simulink model "MultiAgent"  (R2021b)
settings: Solver=ode3  StartTime=0.0  StopTime=160  FixedStep=Ts  RelTol=1e-3
values from neighbouring files (symbols this model uses):
  inner_h = 0.1    [dataset.mat]    (also in initiateVars.m; system_workspace.mat; system_workspace_ayk.mat)
  omega_max_lim = 2500    [dataset.mat]    (also in initiateVars.m; system_workspace.mat; system_workspace_ayk.mat)
  omega_min_lim = 0    [dataset.mat]    (also in initiateVars.m; system_workspace.mat; system_workspace_ayk.mat)
  T_max_lim = 0.495    [dataset.mat]    (also in initiateVars.m = Tp - (Tp - Tm) * sat_lim; system_workspace.mat; system_workspace_ayk.mat)
  T_min_lim = 0.055    [dataset.mat]    (also in initiateVars.m = Tm + (Tp - Tm) * sat_lim; system_workspace.mat; system_workspace_ayk.mat)
  tau_max_lim = 1e-05    [dataset.mat]    (also in initiateVars.m; system_workspace.mat; system_workspace_ayk.mat)
  tau_min_lim = -1e-05    [dataset.mat]    (also in initiateVars.m; system_workspace.mat; system_workspace_ayk.mat)
libraries: slpidlib x4, robotcorelib x2, uavutilslib x2
settings Model: Creator=aykut  LastModifiedBy=fethi
settings SolverCC: AlgebraicLoopSolver=TrustRegion
settings DataIOCC: ReturnWorkspaceOutputs=off
settings DebuggingCC: SFMachineParentedDataDiag=warning  ArithmeticOperatorsInVariantConditions=warning
settings SFSimCC: CustomCodeUndefinedFunction=UseInterfaceOnly

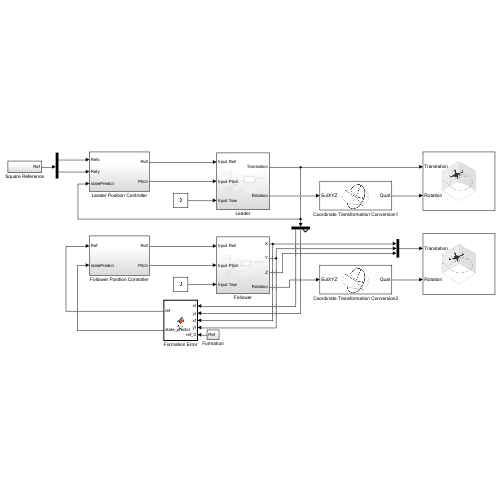
[thumbnail: Simulink's stored preview of the top-level diagram]
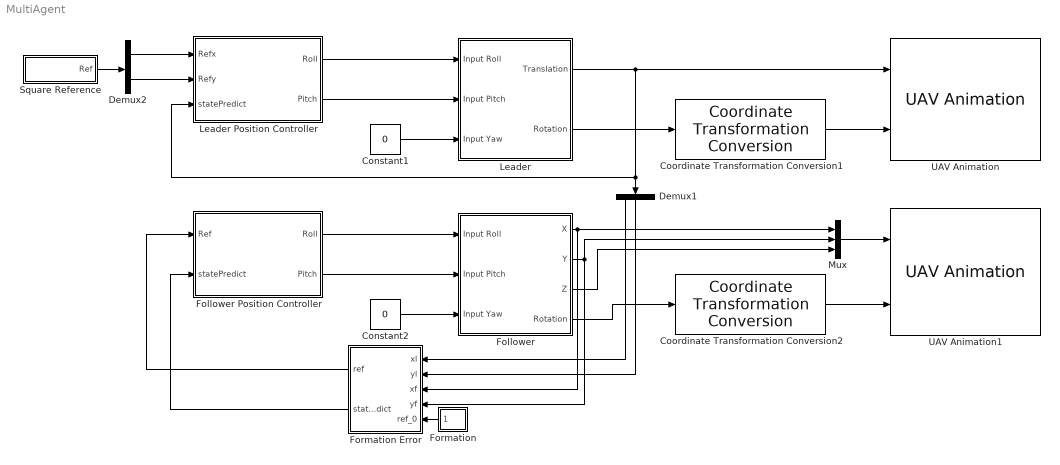
== system MultiAgent ==
  Constant1 : Constant  Value=0
  Constant2 : Constant  Value=0
  Coordinate Transformation Conversion1 : robotcorelib/Coordinate Transformation Conversion  InputRepresentation=Euler Angles  InputEulerSequence=XYZ  ShowTrVecInputPort=on  OutputRepresentation=Quaternion  OutputEulerSequence=ZYX  ShowTrVecOutputPort=on  SimulateUsing=Interpreted execution
      settings: SourceProductBaseCode=NV,RO,RR,UV
  Coordinate Transformation Conversion2 : robotcorelib/Coordinate Transformation Conversion  InputRepresentation=Euler Angles  InputEulerSequence=XYZ  ShowTrVecInputPort=on  OutputRepresentation=Quaternion  OutputEulerSequence=ZYX  ShowTrVecOutputPort=on  SimulateUsing=Interpreted execution
      settings: SourceProductBaseCode=NV,RO,RR,UV
  Demux1 : Demux  Outputs=3
  Demux2 : Demux  Outputs=2
  Follower : Subsystem
  Follower Position Controller : Subsystem
  Formation : Subsystem
  Formation Error : MATLAB Function  TreatAsAtomicUnit=on
  Leader : Subsystem
  Leader Position Controller : Subsystem
  Mux : Mux  Inputs=3
  Square Reference : Subsystem
  UAV Animation : uavutilslib/UAV Animation  UAVType=Multirotor  UAVSize=0.5  InertialZDirection=Up  SampleTime=-1
      settings: SourceProductBaseCode=UV
  UAV Animation1 : uavutilslib/UAV Animation  UAVType=Multirotor  UAVSize=0.5  InertialZDirection=Up  SampleTime=-1
      settings: SourceProductBaseCode=UV
  wires:
  Leader/1(Translation) -> Demux1/1, Leader Position Controller/3(statePredict), UAV Animation/1
  Follower/1(X) -> Formation Error/3(xf), Mux/1
  Follower/2(Y) -> Formation Error/4(yf), Mux/2
  Constant1/1 -> Leader/3(Input Yaw)
  Follower Position Controller/2(Pitch) -> Follower/2(Input Pitch)
  Follower Position Controller/1(Roll) -> Follower/1(Input Roll)
  Constant2/1 -> Follower/3(Input Yaw)
  Leader Position Controller/1(Roll) -> Leader/1(Input Roll)
  Leader Position Controller/2(Pitch) -> Leader/2(Input Pitch)
  Demux2/1 -> Leader Position Controller/1(Refx)
  Demux2/2 -> Leader Position Controller/2(Refy)
  Leader/2(Rotation) -> Coordinate Transformation Conversion1/1
  Coordinate Transformation Conversion1/1 -> UAV Animation/2
  Demux1/1 -> Formation Error/1(xl)
  Demux1/2 -> Formation Error/2(yl)
  Coordinate Transformation Conversion2/1 -> UAV Animation1/2
  Follower/4(Rotation) -> Coordinate Transformation Conversion2/1
  Mux/1 -> UAV Animation1/1
  Square Reference/1(Ref) -> Demux2/1
  Formation Error/1(ref) -> Follower Position Controller/1(Ref)
  Follower/3(Z) -> Mux/3
  Formation Error/2(state_predict) -> Follower Position Controller/2(statePredict)
  Formation/1(Ref) -> Formation Error/5(ref_0)

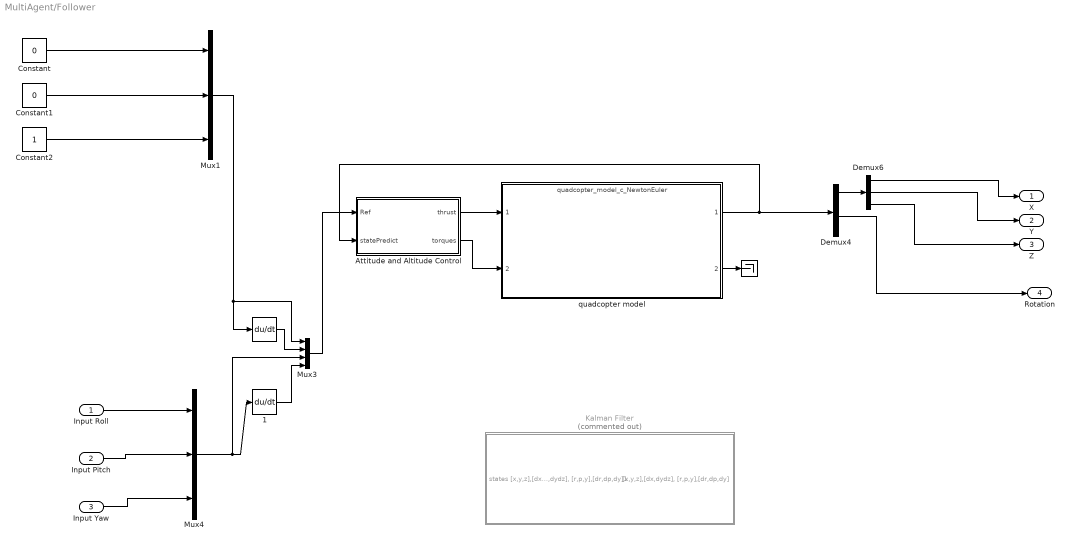
== system MultiAgent/Follower ==
  Input Roll : Inport
  Input Pitch : Inport  Port=2
  Input Yaw : Inport  Port=3
  "   " : Terminator
  "        " : Derivative
  "        1" : Derivative
  Attitude and Altitude Control : Subsystem
  Constant : Constant  Value=0
  Constant1 : Constant  Value=0
  Constant2 : Constant
  Demux4 : Demux  Outputs=[3,3,3,3]
  Demux6 : Demux  Outputs=[1,1,1]
  Kalman Filter : Subsystem  Commented=on
  Mux1 : Mux  Inputs=3
  Mux3 : Mux
  Mux4 : Mux  Inputs=3
  quadcopter model : ModelReference  ModelNameDialog=quadcopter_model_c_NewtonEuler.mdl  SimulationMode=Normal  ModelReferenceVersion=1.355
  X : Outport
  Y : Outport  Port=2
  Z : Outport  Port=3
  Rotation : Outport  Port=4
  wires:
  Mux4/1 -> Mux3/3, "        1"/1
  "        1"/1 -> Mux3/4
  Mux3/1 -> Attitude and Altitude Control/1(Ref)
  Constant/1 -> Mux1/1
  Constant1/1 -> Mux1/2
  "        "/1 -> Mux3/2
  Input Roll/1 -> Mux4/1
  Input Yaw/1 -> Mux4/3
  Constant2/1 -> Mux1/3
  Input Pitch/1 -> Mux4/2
  Mux1/1 -> "        "/1, Mux3/1
  Demux4/1 -> Demux6/1
  quadcopter model/1 -> Attitude and Altitude Control/2(statePredict), Demux4/1
  Attitude and Altitude Control/1(thrust) -> quadcopter model/1
  quadcopter model/2 -> "   "/1
  Attitude and Altitude Control/2(torques) -> quadcopter model/2
  Demux6/1 -> X/1
  Demux6/2 -> Y/1
  Demux6/3 -> Z/1
  Demux4/3 -> Rotation/1

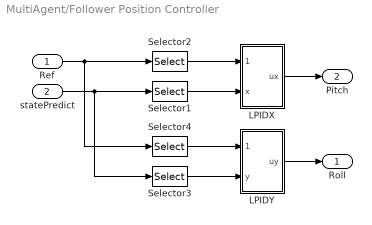
== system MultiAgent/Follower Position Controller ==
  Ref : Inport
  statePredict : Inport  Port=2
  LPIDX : Subsystem
  LPIDY : Subsystem
  Selector1 : Selector  InputPortWidth=2  IndexOptions=Index vector (dialog)  Indices=1  OutputSizes=1
  Selector2 : Selector  InputPortWidth=2  IndexOptions=Index vector (dialog)  Indices=1  OutputSizes=1
  Selector3 : Selector  InputPortWidth=2  IndexOptions=Index vector (dialog)  Indices=2  OutputSizes=1
  Selector4 : Selector  InputPortWidth=2  IndexOptions=Index vector (dialog)  Indices=2  OutputSizes=1
  Roll : Outport  VectorParamsAs1DForOutWhenUnconnected=off
  Pitch : Outport  Port=2  VectorParamsAs1DForOutWhenUnconnected=off
  wires:
  LPIDX/1(ux) -> Pitch/1
  LPIDY/1(uy) -> Roll/1
  statePredict/1 -> Selector1/1, Selector3/1
  Selector3/1 -> LPIDY/2(y)
  Selector1/1 -> LPIDX/2(x)
  Selector2/1 -> LPIDX/1(Refx)
  Ref/1 -> Selector4/1, Selector2/1
  Selector4/1 -> LPIDY/1(Refy)

== system MultiAgent/Formation ==
  Clock : Clock
      settings: Decimation=110
  Mux : Mux  Inputs=2
  Refence Source : MATLAB Function  TreatAsAtomicUnit=on
  Ref : Outport  VectorParamsAs1DForOutWhenUnconnected=off
  wires:
  Refence Source/2(ref_Y) -> Mux/2
  Refence Source/1(ref_X) -> Mux/1
  Mux/1 -> Ref/1
  Clock/1 -> Refence Source/1(timer)

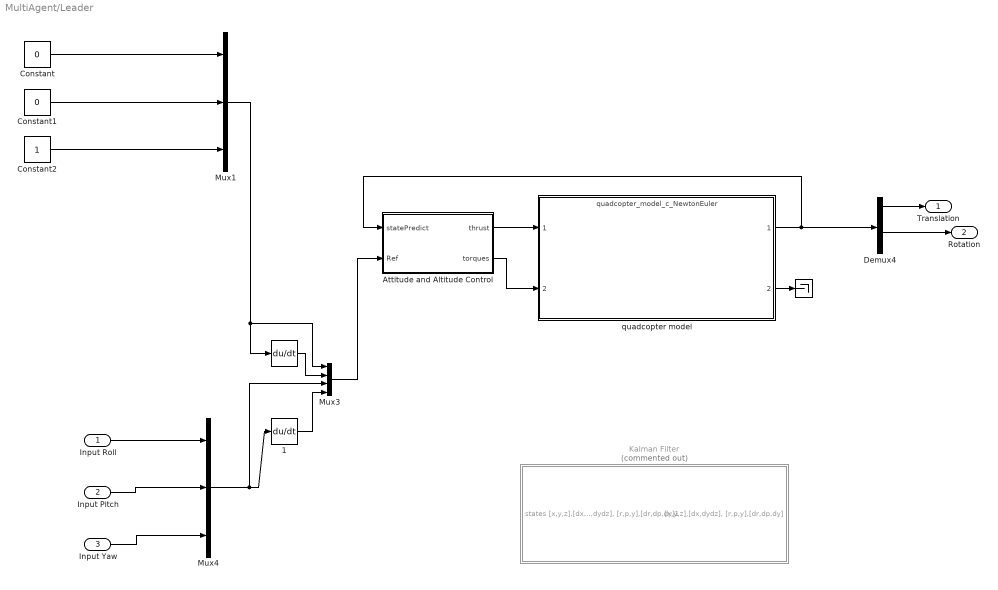
== system MultiAgent/Leader ==
  Input Roll : Inport
  Input Pitch : Inport  Port=2
  Input Yaw : Inport  Port=3
  "   " : Terminator
  "        " : Derivative
  "        1" : Derivative
  Attitude and Altitude Control : Subsystem
  Constant : Constant  Value=0
  Constant1 : Constant  Value=0
  Constant2 : Constant
  Demux4 : Demux  Outputs=[3,3,3,3]
  Kalman Filter : Subsystem  Commented=on
  Mux1 : Mux  Inputs=3
  Mux3 : Mux
  Mux4 : Mux  Inputs=3
  quadcopter model : ModelReference  ModelNameDialog=quadcopter_model_c_NewtonEuler.mdl  SimulationMode=Normal  ModelReferenceVersion=1.355
  Translation : Outport
  Rotation : Outport  Port=2
  wires:
  Attitude and Altitude Control/2(torques) -> quadcopter model/2
  quadcopter model/2 -> "   "/1
  Attitude and Altitude Control/1(thrust) -> quadcopter model/1
  Mux1/1 -> Mux3/1, "        "/1
  Input Pitch/1 -> Mux4/2
  Constant2/1 -> Mux1/3
  Input Yaw/1 -> Mux4/3
  Input Roll/1 -> Mux4/1
  "        "/1 -> Mux3/2
  Constant1/1 -> Mux1/2
  Constant/1 -> Mux1/1
  Mux3/1 -> Attitude and Altitude Control/2(Ref)
  "        1"/1 -> Mux3/4
  Mux4/1 -> "        1"/1, Mux3/3
  quadcopter model/1 -> Attitude and Altitude Control/1(statePredict), Demux4/1
  Demux4/1 -> Translation/1
  Demux4/3 -> Rotation/1

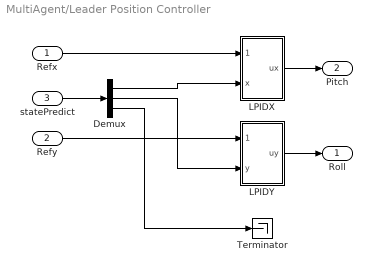
== system MultiAgent/Leader Position Controller ==
  Refx : Inport
  Refy : Inport  Port=2
  statePredict : Inport  Port=3
  Demux : Demux  Outputs=3
  LPIDX : Subsystem
  LPIDY : Subsystem
  Terminator : Terminator
  Roll : Outport  VectorParamsAs1DForOutWhenUnconnected=off
  Pitch : Outport  Port=2  VectorParamsAs1DForOutWhenUnconnected=off
  wires:
  Refx/1 -> LPIDX/1(Refx)
  Refy/1 -> LPIDY/1(Refy)
  LPIDY/1(uy) -> Roll/1
  LPIDX/1(ux) -> Pitch/1
  statePredict/1 -> Demux/1
  Demux/1 -> LPIDX/2(x)
  Demux/2 -> LPIDY/2(y)
  Demux/3 -> Terminator/1

== system MultiAgent/Square Reference ==
  Clock : Clock
      settings: Decimation=110
  Mux : Mux  Inputs=2
  Refence Source : MATLAB Function  TreatAsAtomicUnit=on
  Ref : Outport  VectorParamsAs1DForOutWhenUnconnected=off
  wires:
  Clock/1 -> Refence Source/1(timer)
  Mux/1 -> Ref/1
  Refence Source/1(ref_X) -> Mux/1
  Refence Source/2(ref_Y) -> Mux/2

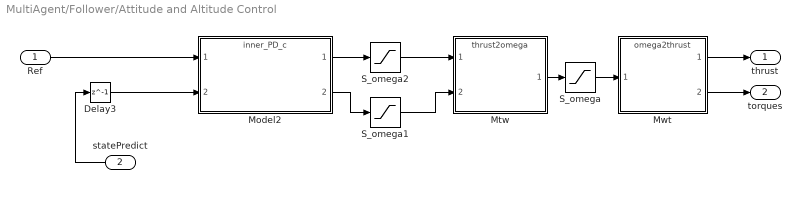
== system MultiAgent/Follower/Attitude and Altitude Control ==
  Ref : Inport
  statePredict : Inport  Port=2
  Delay3 : Delay  DelayLength=1  InitialCondition=0  SampleTime=inner_h
  Model2 : ModelReference  ModelNameDialog=inner_PD_c.mdl  SimulationMode=Normal  ModelReferenceVersion=1.90
  Mtw : ModelReference  ModelNameDialog=thrust2omega.mdl  SimulationMode=Normal  ModelReferenceVersion=1.7
  Mwt : ModelReference  ModelNameDialog=omega2thrust.mdl  SimulationMode=Normal  ModelReferenceVersion=1.7
  S_omega : Saturate  UpperLimit=omega_max_lim  LowerLimit=omega_min_lim
  S_omega1 : Saturate  UpperLimit=tau_max_lim  LowerLimit=tau_min_lim
  S_omega2 : Saturate  UpperLimit=T_max_lim  LowerLimit=T_min_lim
  thrust : Outport  VectorParamsAs1DForOutWhenUnconnected=off
  torques : Outport  Port=2  VectorParamsAs1DForOutWhenUnconnected=off
  wires:
  S_omega/1 -> Mwt/1
  S_omega1/1 -> Mtw/2
  S_omega2/1 -> Mtw/1
  Mtw/1 -> S_omega/1
  Model2/1 -> S_omega2/1
  Mwt/1 -> thrust/1
  Model2/2 -> S_omega1/1
  Delay3/1 -> Model2/2
  Ref/1 -> Model2/1
  Mwt/2 -> torques/1
  statePredict/1 -> Delay3/1

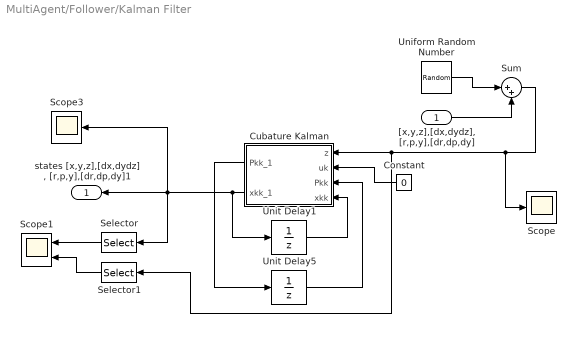
== system MultiAgent/Follower/Kalman Filter ==
  "[x,y,z],[dx,dydz], [r,p,y],[dr,dp,dy]" : Inport
  Constant : Constant  Value=0
  Cubature Kalman : MATLAB Function  TreatAsAtomicUnit=on
  Scope : Scope
  Scope1 : Scope  NumInputPorts=2
  Scope3 : Scope
  Selector : Selector  InputPortWidth=12  IndexOptions=Index vector (dialog)  Indices=[3]  OutputSizes=1
  Selector1 : Selector  InputPortWidth=12  IndexOptions=Index vector (dialog)  Indices=[3]  OutputSizes=1
  Sum : Sum  Inputs=|++
  Uniform Random Number : UniformRandomNumber  Minimum=-0.001  Maximum=0.001  SampleTime=0.1
  Unit Delay1 : UnitDelay  InitialCondition=[0 0 0 0 0 0 0 0 0 0 0 0]  SampleTime=-1  HasFrameUpgradeWarning=on
  Unit Delay5 : UnitDelay  InitialCondition=eye(12)*10^-3  SampleTime=-1  HasFrameUpgradeWarning=on
  "states [x,y,z],[dx,dydz], [r,p,y],[dr,dp,dy]1" : Outport  PortDimensions=12  VectorParamsAs1DForOutWhenUnconnected=off
  wires:
  Unit Delay5/1 -> Cubature Kalman/3(Pkk)
  Cubature Kalman/1(Pkk_1) -> Unit Delay5/1
  Constant/1 -> Cubature Kalman/2(uk)
  Cubature Kalman/2(xkk_1) -> Selector/1, "states [x,y,z],[dx,dydz], [r,p,y],[dr,dp,dy]1"/1, Scope3/1, Unit Delay1/1
  Unit Delay1/1 -> Cubature Kalman/4(xkk)
  Selector/1 -> Scope1/1
  Selector1/1 -> Scope1/2
  Sum/1 -> Selector1/1, Cubature Kalman/1(z), Scope/1
  Uniform Random Number/1 -> Sum/1
  "[x,y,z],[dx,dydz], [r,p,y],[dr,dp,dy]"/1 -> Sum/2

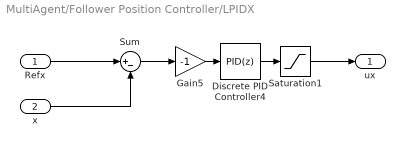
== system MultiAgent/Follower Position Controller/LPIDX ==
  Refx : Inport
  x : Inport  Port=2
  Discrete PID Controller4 : slpidlib/PID Controller  Controller=PID  Form=Parallel  TimeDomain=Discrete-time  UseExternalTs=off  SampleTime=-1  IntegratorMethod=Forward Euler  FilterMethod=Forward Euler  ControllerParametersSource=internal  P=-0.034  I=-8.37942170328314e-06  D=-0.0838262219971284  UseFilter=on  N=16.4387565401463  TunerSelectOption=Transfer Function Based (PID Tuner App)  InitialConditionSource=internal  InitialConditionForIntegrator=0  InitialConditionForFilter=0  DifferentiatorICPrevScaledInput=0  ExternalReset=none  TrackingMode=off  Kt=1  LimitOutput=off  SatLimitsSource=internal  UpperSaturationLimit=inf  LowerSaturationLimit=-inf  LinearizeAsGain=off  AntiWindupMode=none  Kb=1  POutMin=[]  POutMax=[]  IOutMin=[]  IOutMax=[]  DOutMin=[]  DOutMax=[]  NOutMin=[]  NOutMax=[]  SumOutMin=[]  SumOutMax=[]  SaturationOutMin=[]  SaturationOutMax=[]  PParamMin=[]  PParamMax=[]  IParamMin=[]  IParamMax=[]  DParamMin=[]  DParamMax=[]  NParamMin=[]  NParamMax=[]  KbParamMin=[]  KbParamMax=[]  KtParamMin=[]  KtParamMax=[]  KbOutMin=[]  KbOutMax=[]  KtOutMin=[]  KtOutMax=[]  IntegratorOutMin=[]  IntegratorOutMax=[]  FilterOutMin=[]  FilterOutMax=[]  SumI1OutMin=[]  SumI1OutMax=[]  SumI2OutMin=[]  SumI2OutMax=[]  SumI3OutMin=[]  SumI3OutMax=[]  SumI4OutMin=[]  SumI4OutMax=[]  SumDOutMin=[]  SumDOutMax=[]  DifferentiatorOutMin=[]  DifferentiatorOutMax=[]  FilterDiffOutCoefMin=[]  FilterDiffOutCoefMax=[]  ReciprocalOutMin=[]  ReciprocalOutMax=[]  SumDenOutMin=[]  SumDenOutMax=[]  SumNumOutMin=[]  SumNumOutMax=[]  DivideOutMin=[]  DivideOutMax=[]  UdiffTsProdOutMin=[]  UdiffTsProdOutMax=[]  NTsProdOutMin=[]  NTsProdOutMax=[]  UintegralTsProdOutMin=[]  UintegralTsProdOutMax=[]  UngainTsProdOutMin=[]  UngainTsProdOutMax=[]  IntegratorContinuousStateAttributes=''  IntegratorStateMustResolveToSignalObject=off  IntegratorRTWStateStorageClass=Auto  FilterContinuousStateAttributes=''  FilterStateMustResolveToSignalObject=off  FilterRTWStateStorageClass=Auto  ParallelPVariant=InternalParameters  IdealPVariant=Disabled  IVariant=InternalParameters  DVariant=InternalParameters  IntegratorVariant=Discrete  SatVariant=Disabled  AWVariant=Passthrough  PCopyVariant=Disabled  TRVariant=Disabled  FdbkBlocksVariant=Forward  IdealPFdbkVariant=Disabled  SatFdbkVariant=Disabled  DerivativeFilterVariant=ForwardEulerFilter  NVariant=InternalParameters  NCopyVariant=Disabled  FilterICVariant=InternalICsFilter  IntegratorICVariant=InternalICs  ExternalResetVariant=Disabled  TRSumVariant=Passthrough  SumFdbkVariant=Disabled  SumVariant=Sum_PID  TsampFilterVariant=InternalTs  TsampNgainVariant=Passthrough  TsampIntegralVariant=Passthrough  ExternalSaturationOutDataTypeStr=Inherit: Same as second input
  Gain5 : Gain  Gain=-1
  Saturation1 : Saturate  UpperLimit=pi/18  LowerLimit=-pi/18
  Sum : Sum  Inputs=|+-
  ux : Outport  VectorParamsAs1DForOutWhenUnconnected=off
  wires:
  Saturation1/1 -> ux/1
  Sum/1 -> Gain5/1
  Discrete PID Controller4/1 -> Saturation1/1
  x/1 -> Sum/2
  Refx/1 -> Sum/1
  Gain5/1 -> Discrete PID Controller4/1

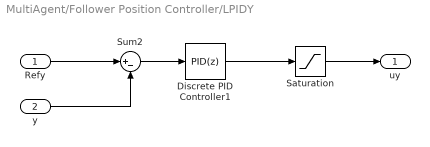
== system MultiAgent/Follower Position Controller/LPIDY ==
  Refy : Inport
  y : Inport  Port=2
  Discrete PID Controller1 : slpidlib/PID Controller  Controller=PID  Form=Parallel  TimeDomain=Discrete-time  UseExternalTs=off  SampleTime=-1  IntegratorMethod=Forward Euler  FilterMethod=Forward Euler  ControllerParametersSource=internal  P=-0.034  I=-8.37942170328314e-06  D=-0.0838262219971284  UseFilter=on  N=16.4387565401463  TunerSelectOption=Transfer Function Based (PID Tuner App)  InitialConditionSource=internal  InitialConditionForIntegrator=0  InitialConditionForFilter=0  DifferentiatorICPrevScaledInput=0  ExternalReset=none  TrackingMode=off  Kt=1  LimitOutput=off  SatLimitsSource=internal  UpperSaturationLimit=inf  LowerSaturationLimit=-inf  LinearizeAsGain=off  AntiWindupMode=none  Kb=1  POutMin=[]  POutMax=[]  IOutMin=[]  IOutMax=[]  DOutMin=[]  DOutMax=[]  NOutMin=[]  NOutMax=[]  SumOutMin=[]  SumOutMax=[]  SaturationOutMin=[]  SaturationOutMax=[]  PParamMin=[]  PParamMax=[]  IParamMin=[]  IParamMax=[]  DParamMin=[]  DParamMax=[]  NParamMin=[]  NParamMax=[]  KbParamMin=[]  KbParamMax=[]  KtParamMin=[]  KtParamMax=[]  KbOutMin=[]  KbOutMax=[]  KtOutMin=[]  KtOutMax=[]  IntegratorOutMin=[]  IntegratorOutMax=[]  FilterOutMin=[]  FilterOutMax=[]  SumI1OutMin=[]  SumI1OutMax=[]  SumI2OutMin=[]  SumI2OutMax=[]  SumI3OutMin=[]  SumI3OutMax=[]  SumI4OutMin=[]  SumI4OutMax=[]  SumDOutMin=[]  SumDOutMax=[]  DifferentiatorOutMin=[]  DifferentiatorOutMax=[]  FilterDiffOutCoefMin=[]  FilterDiffOutCoefMax=[]  ReciprocalOutMin=[]  ReciprocalOutMax=[]  SumDenOutMin=[]  SumDenOutMax=[]  SumNumOutMin=[]  SumNumOutMax=[]  DivideOutMin=[]  DivideOutMax=[]  UdiffTsProdOutMin=[]  UdiffTsProdOutMax=[]  NTsProdOutMin=[]  NTsProdOutMax=[]  UintegralTsProdOutMin=[]  UintegralTsProdOutMax=[]  UngainTsProdOutMin=[]  UngainTsProdOutMax=[]  IntegratorContinuousStateAttributes=''  IntegratorStateMustResolveToSignalObject=off  IntegratorRTWStateStorageClass=Auto  FilterContinuousStateAttributes=''  FilterStateMustResolveToSignalObject=off  FilterRTWStateStorageClass=Auto  ParallelPVariant=InternalParameters  IdealPVariant=Disabled  IVariant=InternalParameters  DVariant=InternalParameters  IntegratorVariant=Discrete  SatVariant=Disabled  AWVariant=Passthrough  PCopyVariant=Disabled  TRVariant=Disabled  FdbkBlocksVariant=Forward  IdealPFdbkVariant=Disabled  SatFdbkVariant=Disabled  DerivativeFilterVariant=ForwardEulerFilter  NVariant=InternalParameters  NCopyVariant=Disabled  FilterICVariant=InternalICsFilter  IntegratorICVariant=InternalICs  ExternalResetVariant=Disabled  TRSumVariant=Passthrough  SumFdbkVariant=Disabled  SumVariant=Sum_PID  TsampFilterVariant=InternalTs  TsampNgainVariant=Passthrough  TsampIntegralVariant=Passthrough  ExternalSaturationOutDataTypeStr=Inherit: Same as second input
  Saturation : Saturate  UpperLimit=pi/18  LowerLimit=-pi/18
  Sum2 : Sum  Inputs=|+-
  uy : Outport  VectorParamsAs1DForOutWhenUnconnected=off
  wires:
  Saturation/1 -> uy/1
  y/1 -> Sum2/2
  Refy/1 -> Sum2/1
  Discrete PID Controller1/1 -> Saturation/1
  Sum2/1 -> Discrete PID Controller1/1

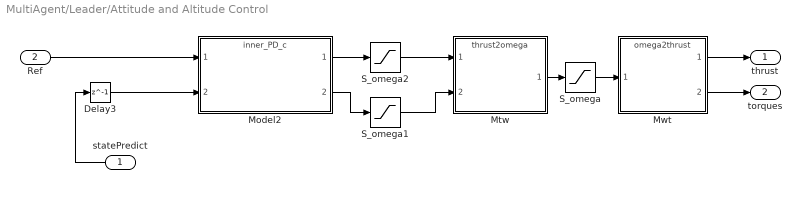
== system MultiAgent/Leader/Attitude and Altitude Control ==
  statePredict : Inport
  Ref : Inport  Port=2
  Delay3 : Delay  DelayLength=1  InitialCondition=0  SampleTime=inner_h
  Model2 : ModelReference  ModelNameDialog=inner_PD_c.mdl  SimulationMode=Normal  ModelReferenceVersion=1.90
  Mtw : ModelReference  ModelNameDialog=thrust2omega.mdl  SimulationMode=Normal  ModelReferenceVersion=1.7
  Mwt : ModelReference  ModelNameDialog=omega2thrust.mdl  SimulationMode=Normal  ModelReferenceVersion=1.7
  S_omega : Saturate  UpperLimit=omega_max_lim  LowerLimit=omega_min_lim
  S_omega1 : Saturate  UpperLimit=tau_max_lim  LowerLimit=tau_min_lim
  S_omega2 : Saturate  UpperLimit=T_max_lim  LowerLimit=T_min_lim
  thrust : Outport  VectorParamsAs1DForOutWhenUnconnected=off
  torques : Outport  Port=2  VectorParamsAs1DForOutWhenUnconnected=off
  wires:
  statePredict/1 -> Delay3/1
  Mwt/2 -> torques/1
  Ref/1 -> Model2/1
  Delay3/1 -> Model2/2
  Model2/2 -> S_omega1/1
  Mwt/1 -> thrust/1
  Model2/1 -> S_omega2/1
  Mtw/1 -> S_omega/1
  S_omega2/1 -> Mtw/1
  S_omega1/1 -> Mtw/2
  S_omega/1 -> Mwt/1

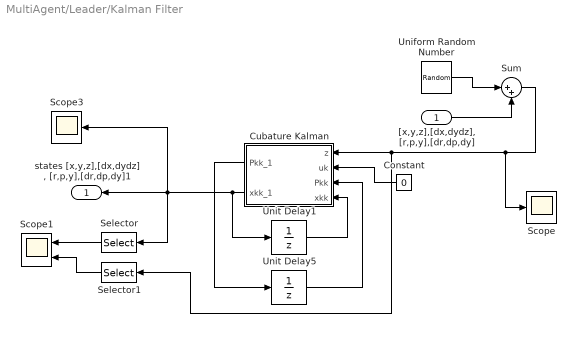
== system MultiAgent/Leader/Kalman Filter ==
  "[x,y,z],[dx,dydz], [r,p,y],[dr,dp,dy]" : Inport
  Constant : Constant  Value=0
  Cubature Kalman : MATLAB Function  TreatAsAtomicUnit=on
  Scope : Scope
  Scope1 : Scope  NumInputPorts=2
  Scope3 : Scope
  Selector : Selector  InputPortWidth=12  IndexOptions=Index vector (dialog)  Indices=[3]  OutputSizes=1
  Selector1 : Selector  InputPortWidth=12  IndexOptions=Index vector (dialog)  Indices=[3]  OutputSizes=1
  Sum : Sum  Inputs=|++
  Uniform Random Number : UniformRandomNumber  Minimum=-0.001  Maximum=0.001  SampleTime=0.1
  Unit Delay1 : UnitDelay  InitialCondition=[0 0 0 0 0 0 0 0 0 0 0 0]  SampleTime=-1  HasFrameUpgradeWarning=on
  Unit Delay5 : UnitDelay  InitialCondition=eye(12)*10^-3  SampleTime=-1  HasFrameUpgradeWarning=on
  "states [x,y,z],[dx,dydz], [r,p,y],[dr,dp,dy]1" : Outport  PortDimensions=12  VectorParamsAs1DForOutWhenUnconnected=off
  wires:
  "[x,y,z],[dx,dydz], [r,p,y],[dr,dp,dy]"/1 -> Sum/2
  Uniform Random Number/1 -> Sum/1
  Sum/1 -> Scope/1, Cubature Kalman/1(z), Selector1/1
  Selector1/1 -> Scope1/2
  Selector/1 -> Scope1/1
  Unit Delay1/1 -> Cubature Kalman/4(xkk)
  Cubature Kalman/2(xkk_1) -> Unit Delay1/1, Scope3/1, "states [x,y,z],[dx,dydz], [r,p,y],[dr,dp,dy]1"/1, Selector/1
  Constant/1 -> Cubature Kalman/2(uk)
  Cubature Kalman/1(Pkk_1) -> Unit Delay5/1
  Unit Delay5/1 -> Cubature Kalman/3(Pkk)

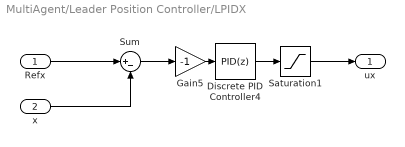
== system MultiAgent/Leader Position Controller/LPIDX ==
  Refx : Inport
  x : Inport  Port=2
  Discrete PID Controller4 : slpidlib/PID Controller  Controller=PID  Form=Parallel  TimeDomain=Discrete-time  UseExternalTs=off  SampleTime=-1  IntegratorMethod=Forward Euler  FilterMethod=Forward Euler  ControllerParametersSource=internal  P=-0.034  I=-7.00942170328314e-06  D=-0.0838262219971284  UseFilter=on  N=16.4387565401463  TunerSelectOption=Transfer Function Based (PID Tuner App)  InitialConditionSource=internal  InitialConditionForIntegrator=0  InitialConditionForFilter=0  DifferentiatorICPrevScaledInput=0  ExternalReset=none  TrackingMode=off  Kt=1  LimitOutput=off  SatLimitsSource=internal  UpperSaturationLimit=inf  LowerSaturationLimit=-inf  LinearizeAsGain=off  AntiWindupMode=none  Kb=1  POutMin=[]  POutMax=[]  IOutMin=[]  IOutMax=[]  DOutMin=[]  DOutMax=[]  NOutMin=[]  NOutMax=[]  SumOutMin=[]  SumOutMax=[]  SaturationOutMin=[]  SaturationOutMax=[]  PParamMin=[]  PParamMax=[]  IParamMin=[]  IParamMax=[]  DParamMin=[]  DParamMax=[]  NParamMin=[]  NParamMax=[]  KbParamMin=[]  KbParamMax=[]  KtParamMin=[]  KtParamMax=[]  KbOutMin=[]  KbOutMax=[]  KtOutMin=[]  KtOutMax=[]  IntegratorOutMin=[]  IntegratorOutMax=[]  FilterOutMin=[]  FilterOutMax=[]  SumI1OutMin=[]  SumI1OutMax=[]  SumI2OutMin=[]  SumI2OutMax=[]  SumI3OutMin=[]  SumI3OutMax=[]  SumI4OutMin=[]  SumI4OutMax=[]  SumDOutMin=[]  SumDOutMax=[]  DifferentiatorOutMin=[]  DifferentiatorOutMax=[]  FilterDiffOutCoefMin=[]  FilterDiffOutCoefMax=[]  ReciprocalOutMin=[]  ReciprocalOutMax=[]  SumDenOutMin=[]  SumDenOutMax=[]  SumNumOutMin=[]  SumNumOutMax=[]  DivideOutMin=[]  DivideOutMax=[]  UdiffTsProdOutMin=[]  UdiffTsProdOutMax=[]  NTsProdOutMin=[]  NTsProdOutMax=[]  UintegralTsProdOutMin=[]  UintegralTsProdOutMax=[]  UngainTsProdOutMin=[]  UngainTsProdOutMax=[]  IntegratorContinuousStateAttributes=''  IntegratorStateMustResolveToSignalObject=off  IntegratorRTWStateStorageClass=Auto  FilterContinuousStateAttributes=''  FilterStateMustResolveToSignalObject=off  FilterRTWStateStorageClass=Auto  ParallelPVariant=InternalParameters  IdealPVariant=Disabled  IVariant=InternalParameters  DVariant=InternalParameters  IntegratorVariant=Discrete  SatVariant=Disabled  AWVariant=Passthrough  PCopyVariant=Disabled  TRVariant=Disabled  FdbkBlocksVariant=Forward  IdealPFdbkVariant=Disabled  SatFdbkVariant=Disabled  DerivativeFilterVariant=ForwardEulerFilter  NVariant=InternalParameters  NCopyVariant=Disabled  FilterICVariant=InternalICsFilter  IntegratorICVariant=InternalICs  ExternalResetVariant=Disabled  TRSumVariant=Passthrough  SumFdbkVariant=Disabled  SumVariant=Sum_PID  TsampFilterVariant=InternalTs  TsampNgainVariant=Passthrough  TsampIntegralVariant=Passthrough  ExternalSaturationOutDataTypeStr=Inherit: Same as second input
  Gain5 : Gain  Gain=-1
  Saturation1 : Saturate  UpperLimit=pi/18  LowerLimit=-pi/18
  Sum : Sum  Inputs=|+-
  ux : Outport  VectorParamsAs1DForOutWhenUnconnected=off
  wires:
  Refx/1 -> Sum/1
  x/1 -> Sum/2
  Discrete PID Controller4/1 -> Saturation1/1
  Sum/1 -> Gain5/1
  Gain5/1 -> Discrete PID Controller4/1
  Saturation1/1 -> ux/1

== system MultiAgent/Leader Position Controller/LPIDY ==
  Refy : Inport
  y : Inport  Port=2
  Discrete PID Controller1 : slpidlib/PID Controller  Controller=PID  Form=Parallel  TimeDomain=Discrete-time  UseExternalTs=off  SampleTime=-1  IntegratorMethod=Forward Euler  FilterMethod=Forward Euler  ControllerParametersSource=internal  P=-0.034  I=-7.00942170328314e-06  D=-0.0838262219971284  UseFilter=on  N=16.4387565401463  TunerSelectOption=Transfer Function Based (PID Tuner App)  InitialConditionSource=internal  InitialConditionForIntegrator=0  InitialConditionForFilter=0  DifferentiatorICPrevScaledInput=0  ExternalReset=none  TrackingMode=off  Kt=1  LimitOutput=off  SatLimitsSource=internal  UpperSaturationLimit=inf  LowerSaturationLimit=-inf  LinearizeAsGain=off  AntiWindupMode=none  Kb=1  POutMin=[]  POutMax=[]  IOutMin=[]  IOutMax=[]  DOutMin=[]  DOutMax=[]  NOutMin=[]  NOutMax=[]  SumOutMin=[]  SumOutMax=[]  SaturationOutMin=[]  SaturationOutMax=[]  PParamMin=[]  PParamMax=[]  IParamMin=[]  IParamMax=[]  DParamMin=[]  DParamMax=[]  NParamMin=[]  NParamMax=[]  KbParamMin=[]  KbParamMax=[]  KtParamMin=[]  KtParamMax=[]  KbOutMin=[]  KbOutMax=[]  KtOutMin=[]  KtOutMax=[]  IntegratorOutMin=[]  IntegratorOutMax=[]  FilterOutMin=[]  FilterOutMax=[]  SumI1OutMin=[]  SumI1OutMax=[]  SumI2OutMin=[]  SumI2OutMax=[]  SumI3OutMin=[]  SumI3OutMax=[]  SumI4OutMin=[]  SumI4OutMax=[]  SumDOutMin=[]  SumDOutMax=[]  DifferentiatorOutMin=[]  DifferentiatorOutMax=[]  FilterDiffOutCoefMin=[]  FilterDiffOutCoefMax=[]  ReciprocalOutMin=[]  ReciprocalOutMax=[]  SumDenOutMin=[]  SumDenOutMax=[]  SumNumOutMin=[]  SumNumOutMax=[]  DivideOutMin=[]  DivideOutMax=[]  UdiffTsProdOutMin=[]  UdiffTsProdOutMax=[]  NTsProdOutMin=[]  NTsProdOutMax=[]  UintegralTsProdOutMin=[]  UintegralTsProdOutMax=[]  UngainTsProdOutMin=[]  UngainTsProdOutMax=[]  IntegratorContinuousStateAttributes=''  IntegratorStateMustResolveToSignalObject=off  IntegratorRTWStateStorageClass=Auto  FilterContinuousStateAttributes=''  FilterStateMustResolveToSignalObject=off  FilterRTWStateStorageClass=Auto  ParallelPVariant=InternalParameters  IdealPVariant=Disabled  IVariant=InternalParameters  DVariant=InternalParameters  IntegratorVariant=Discrete  SatVariant=Disabled  AWVariant=Passthrough  PCopyVariant=Disabled  TRVariant=Disabled  FdbkBlocksVariant=Forward  IdealPFdbkVariant=Disabled  SatFdbkVariant=Disabled  DerivativeFilterVariant=ForwardEulerFilter  NVariant=InternalParameters  NCopyVariant=Disabled  FilterICVariant=InternalICsFilter  IntegratorICVariant=InternalICs  ExternalResetVariant=Disabled  TRSumVariant=Passthrough  SumFdbkVariant=Disabled  SumVariant=Sum_PID  TsampFilterVariant=InternalTs  TsampNgainVariant=Passthrough  TsampIntegralVariant=Passthrough  ExternalSaturationOutDataTypeStr=Inherit: Same as second input
  Saturation : Saturate  UpperLimit=pi/18  LowerLimit=-pi/18
  Sum2 : Sum  Inputs=|+-
  uy : Outport  VectorParamsAs1DForOutWhenUnconnected=off
  wires:
  Refy/1 -> Sum2/1
  y/1 -> Sum2/2
  Sum2/1 -> Discrete PID Controller1/1
  Saturation/1 -> uy/1
  Discrete PID Controller1/1 -> Saturation/1

== matlab function MultiAgent/Leader/Kalman Filter/Cubature Kalman ==
  data: Pkk_1 output; z input; uk input; Pkk input; xkk input; xkk_1 output
function [Pkk_1, xkk_1]   = fcn(z, uk, Pkk, xkk)

%% Model
A = 1;
B = 0;

%% Covariances
Q = diag([0.1 0.1 0.1 0.1 0.1 0.1 0.1 0.1 0.1 0.1 0.1 0.1])*100;
R = 0.01;   
% gyro = z(4:6);
% delta = [1*(gyro'-xkk(4:6));0;0;0;0];
% z1 = [z(1:3)' - xkk(1:3); z(1:3)' - xkk(1:3); z(7)];  
%% Cubature Kalman Predict
xkk1 = A*xkk ;
Pkk1 = A*Pkk*A' + Q; 

%% Cubature Kalman Update
%%%========================================================================
%%% Genrate a set of Cubature Points
%%%========================================================================

nx = 12; % state vector dimension

nPts = 2*nx;   % No. of Cubature Points

CPtArray = sqrt(nPts/2)*[eye(nx) -eye(nx)];

%%%========================================================================
%%% find the square-root of Pkk1 using Singular Value Decomposition (SVD)
%%%========================================================================

Pkk1 = 0.5*(Pkk1+Pkk1'); % make Pkk1 to be symmetric (Property of a covariance matrix !)

[U, S, V] =  svd(Pkk1);

Skk1 = 0.5*(U+V)*sqrt(S);

%%%========================================================================

Xi =  repmat(xkk1,1,nPts) + Skk1*CPtArray;

% Zi = Zi1(1,:);
% Zi = cartpend(Xi,uk, Zi1);
% bias = [0.00017;0.00017;0.00017;0.00076;0.00076;0.00076;0.001]; 
% bias = repmat(bias,1,14);
Zi = Xi;
% Zi = Zi1';

    

zkk1 = sum(Zi,2)/nPts;      % predicted Measurement

X = (Xi-repmat(xkk1,1,nPts))/sqrt(nPts);
    
Z = (Zi-repmat(zkk1,1,nPts))/sqrt(nPts);  

Pzz = Z*Z'+ R; % Innovations Covariance

Pxz = X*Z'; % cross-covariance
    
G = Pxz*pinv(Pzz);         % Cubature Kalman Gain  
    
xkk_1 = xkk1 + G*(z - zkk1);  

Pkk_1 = Pkk1 - G*Pzz*G';

== matlab function MultiAgent/Follower/Kalman Filter/Cubature Kalman ==
  data: Pkk_1 output; z input; uk input; Pkk input; xkk input; xkk_1 output
function [Pkk_1, xkk_1]   = fcn(z, uk, Pkk, xkk)

%% Model
A = 1;
B = 0;

%% Covariances
Q = diag([0.1 0.1 0.1 0.1 0.1 0.1 0.1 0.1 0.1 0.1 0.1 0.1])*100;
R = 0.01;   
% gyro = z(4:6);
% delta = [1*(gyro'-xkk(4:6));0;0;0;0];
% z1 = [z(1:3)' - xkk(1:3); z(1:3)' - xkk(1:3); z(7)];  
%% Cubature Kalman Predict
xkk1 = A*xkk ;
Pkk1 = A*Pkk*A' + Q; 

%% Cubature Kalman Update
%%%========================================================================
%%% Genrate a set of Cubature Points
%%%========================================================================

nx = 12; % state vector dimension

nPts = 2*nx;   % No. of Cubature Points

CPtArray = sqrt(nPts/2)*[eye(nx) -eye(nx)];

%%%========================================================================
%%% find the square-root of Pkk1 using Singular Value Decomposition (SVD)
%%%========================================================================

Pkk1 = 0.5*(Pkk1+Pkk1'); % make Pkk1 to be symmetric (Property of a covariance matrix !)

[U, S, V] =  svd(Pkk1);

Skk1 = 0.5*(U+V)*sqrt(S);

%%%========================================================================

Xi =  repmat(xkk1,1,nPts) + Skk1*CPtArray;

% Zi = Zi1(1,:);
% Zi = cartpend(Xi,uk, Zi1);
% bias = [0.00017;0.00017;0.00017;0.00076;0.00076;0.00076;0.001]; 
% bias = repmat(bias,1,14);
Zi = Xi;
% Zi = Zi1';

    

zkk1 = sum(Zi,2)/nPts;      % predicted Measurement

X = (Xi-repmat(xkk1,1,nPts))/sqrt(nPts);
    
Z = (Zi-repmat(zkk1,1,nPts))/sqrt(nPts);  

Pzz = Z*Z'+ R; % Innovations Covariance

Pxz = X*Z'; % cross-covariance
    
G = Pxz*pinv(Pzz);         % Cubature Kalman Gain  
    
xkk_1 = xkk1 + G*(z - zkk1);  

Pkk_1 = Pkk1 - G*Pzz*G';

== matlab function MultiAgent/Formation/Refence Source ==
  data: timer input; ref_X output; ref_Y output
function [ref_X,ref_Y] = fcn(timer)

if timer > 0 && timer < 30
    ref_X = 1;
    ref_Y = 1;

elseif timer >= 30 && timer < 50
    ref_X = -1;
    ref_Y = 1;    
  
elseif timer >= 50 && timer < 70
    ref_X = -1;
    ref_Y = -1;  

elseif timer >= 70 && timer < 90
    ref_X = 1;
    ref_Y = -1; 
    
elseif timer >= 90 && timer < 120
    ref_X = 1;
    ref_Y = 1;
else
    ref_X = 1;
    ref_Y = 1;
end

== matlab function MultiAgent/Formation Error ==
  data: ref output; xl input; yl input; xf input; yf input; state_predict output; ref_0 input
function [ref, state_predict]= fcn(xl,yl,xf,yf, ref_0)
yawl = 0;
dx = -(xl - xf)*cosd(yawl) - (yl - yf)*sind(yawl);
dy =  (xl - xf)*sind(yawl) - (yl - yf)*cosd(yawl);
% ref = [-1 1];
ref = ref_0;
state_predict = [dx dy];

% function [refx_f, refy_f, dx, dy]= fcn(xl, yl, xf, yf, platoon)
% 
% heading = atand((yl-yf)/(xl-xf));
% 
% if isnan(heading)
%     heading = 0;
% else
%     heading = heading;
% end
% 
% 
% dx = -(xl - xf)*cosd(heading) - (yl - yf)*sind(heading);
% dy =  (xl - xf)*sind(heading) - (yl - yf)*cosd(heading);
% 
% 
% refx_f = (xl - xf) + platoon;
% refy_f = (yl - yf) + platoon;

% refx_f = 0;
% refy_f = 0;
% 
% distance = sqrt((xl - xf)^2 + (yl - yf)^2);
% error  = platoon - distance;
% 
% if ( sqrt((xl - xf)^2) >= sqrt((yl - yf)^2) )
%     if xl >= xf
%         refx_f = xf - error;
%         refy_f = yf;
%     else
%         refx_f = xf + error;
%         refy_f = yf;
%     end
% else
%     if yl >= yf
%         refy_f = yf - error;
%         refx_f = xf;
%     else
%         refy_f = yf + error;
%         refx_f = xf;
%     end
% end

% if refx_f >= 5
% refx_f = 5;
% else if refx_f <= -5
%     refx_f = -5;
% else
%     refx_f = refx_f;
% end
% 
% if refy_f >= 5
% refy_f = 5;
% else if refy_f <= -5
%     refy_f = -5;
% else
%     refy_f = refy_f;
% end

== matlab function MultiAgent/Square Reference/Refence Source ==
  data: timer input; ref_X output; ref_Y output
function [ref_X,ref_Y] = fcn(timer)

if timer > 0 && timer < 30
    ref_X = 0;
    ref_Y = 0;

elseif timer >= 30 && timer < 50
    ref_X = 5;
    ref_Y = 0;    
  
elseif timer >= 50 && timer < 70
    ref_X = 5;
    ref_Y = 5;  

elseif timer >= 70 && timer < 90
    ref_X = 0;
    ref_Y = 5; 
    
elseif timer >= 90 && timer < 120
    ref_X = 0;
    ref_Y = 0;
else
    ref_X = 0;
    ref_Y = 0;
end
